simulink model "quaternion_differentiation_test"  (R2016a)
settings: Solver=ode4  StartTime=0.0  StopTime=10.0  FixedStep=0.01  RelTol=1e-3
libraries: aerolibtransform2 x3
settings Model: Creator=PD Banneheka  LastModifiedBy=PD Banneheka
settings GRTTargetCC: GeneratePreprocessorConditionals=Use local settings

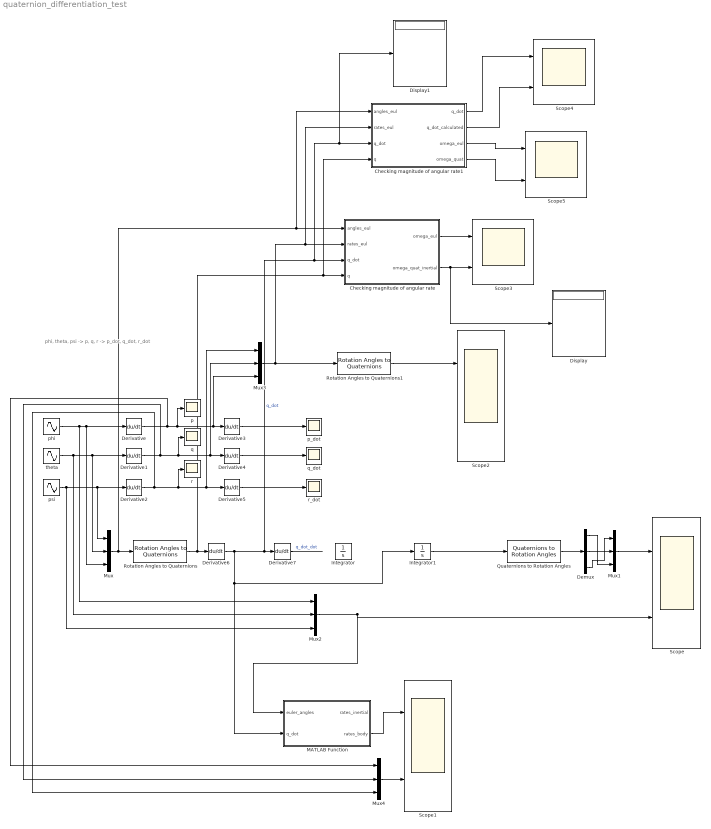
== system quaternion_differentiation_test ==
  note: phi, theta, psi -> p, q, r -> p_dot, q_dot, r_dot
  Checking magnitude of angular rate : MATLAB Function  TreatAsAtomicUnit=on
  Checking magnitude of angular rate1 : MATLAB Function  TreatAsAtomicUnit=on
  Demux : Demux  Outputs=3
  Derivative{,1..7} (8 alike) : Derivative
  Display : Display
  Display1 : Display
  Integrator : Integrator
  Integrator1 : Integrator
  MATLAB Function : MATLAB Function  TreatAsAtomicUnit=on
  Mux{,1..4} (5 alike) : Mux  Inputs=3
  Quaternions to Rotation Angles : aerolibtransform2/Quaternions to Rotation Angles  rotationOrder=ZYX
  Rotation Angles to Quaternions : aerolibtransform2/Rotation Angles to Quaternions  rotationOrder=ZYX
  Rotation Angles to Quaternions1 : aerolibtransform2/Rotation Angles to Quaternions  rotationOrder=ZYX
  Scope{,1..5} (6 alike) : Scope  NumInputPorts=2
  p : Scope
  p_dot : Scope
  phi : Sin  SampleTime=0
  psi : Sin  SampleTime=0
  q : Scope
  q_dot : Scope
  r : Scope
  r_dot : Scope
  theta : Sin  SampleTime=0
  wires:
  phi/1 -> Mux2/1, Mux/3, Derivative/1
  theta/1 -> Mux2/2, Mux/2, Derivative1/1
  psi/1 -> Mux2/3, Derivative2/1, Mux/1
  Derivative3/1 -> p_dot/1
  Derivative4/1 -> q_dot/1
  Derivative5/1 -> r_dot/1
  Mux/1 -> Checking magnitude of angular rate1/1(angles_eul), Checking magnitude of angular rate/1(angles_eul), Rotation Angles to Quaternions/1
  Quaternions to Rotation Angles/1 -> Demux/1
  Demux/1 -> Mux1/3
  Demux/2 -> Mux1/2
  Demux/3 -> Mux1/1
  Mux1/1 -> Scope/1
  Mux2/1 -> MATLAB Function/1(euler_angles), Scope/2
  Mux4/1 -> Scope1/2
  MATLAB Function/2(rates_body) -> Scope1/1
  Derivative/1 -> p/1, Mux3/3, Derivative3/1, Mux4/1
  Derivative1/1 -> q/1, Derivative4/1, Mux3/2, Mux4/2
  Derivative2/1 -> Mux4/3, r/1, Derivative5/1, Mux3/1
  Rotation Angles to Quaternions1/1 -> Scope2/1
  Derivative7/1 -> ?  "q_dot_dot"
  Derivative6/1 -> MATLAB Function/2(q_dot), Integrator1/1, Display1/1, Checking magnitude of angular rate1/3("q_dot "), Checking magnitude of angular rate/3(q_dot), Derivative7/1  "q_dot"
  Rotation Angles to Quaternions/1 -> Derivative6/1, Checking magnitude of angular rate1/4(q), Checking magnitude of angular rate/4(q)
  Integrator1/1 -> Quaternions to Rotation Angles/1
  Mux3/1 -> Checking magnitude of angular rate1/2(rates_eul), Checking magnitude of angular rate/2(rates_eul), Rotation Angles to Quaternions1/1
  Checking magnitude of angular rate/2(omega_quat_inertial) -> Display/1, Scope3/2
  Checking magnitude of angular rate/1(omega_eul) -> Scope3/1
  Checking magnitude of angular rate1/1(q_dot) -> Scope4/1
  Checking magnitude of angular rate1/2(q_dot_calculated) -> Scope4/2
  Checking magnitude of angular rate1/3(omega_eul) -> Scope5/1
  Checking magnitude of angular rate1/4(omega_quat) -> Scope5/2

== matlab function quaternion_differentiation_test/Checking magnitude of angular rate ==
  data: angles_eul input; rates_eul input; omega_eul output; q_dot input; omega_quat_inertial output; q input
function [omega_eul,omega_quat_inertial]= fcn(angles_eul,rates_eul,q_dot,q)
% Checking angular rate
% https://math.stackexchange.com/questions/1792826/estimate-angular-velocity-and-acceleration-from-a-sequence-of-rotations

% Angular rate magnitude using Euler rates
% omega_eul = sqrt(rates_eul(1)^2 + rates_eul(2)^2 + rates_eul(3)^2);
omega_eul = rates_eul;

% From website: omega = 2*q_dot*pinv(q)
% omega_quat = 2*q_dot'*quatinv(q')';
omega_quat = 2*quatmultiply(q_dot',quatinv(q'));

%% Transformation from NASA
% Original axes : inertial/wind/Earth/reference
% Final axes    : body

psi = angles_eul(1); % Yaw angle (first rotation, about z axis)
theta = angles_eul(2); % Pitch angle (second rotation, about y axis)
phi = angles_eul(3); % Roll angle (third rotation, about x axis)

S1 = sin(psi);
C1 = cos(psi);
S2 = sin(theta);
C2 = cos(theta);
S3 = sin(phi);
C3 = cos(phi);
    
M = [   C1*C2               C1*S2*S3-S1*C3      C1*S2*C3+S1*S3
        S1*C2               S1*S2*S3+C1*C3      S1*S2*C3-C1*S3
        -S2                 C2*S3               C2*C3           ]; % x0 = M * x3
    
% omega_quat_inertial = M*omega_quat(2:4)';
omega_quat_inertial = omega_quat(2:4)';

== matlab function quaternion_differentiation_test/MATLAB Function ==
  data: euler_angles input; rates_inertial output; q_dot input; rates_body output
function [rates_inertial,rates_body]= fcn(euler_angles,q_dot)
% From NASA transformation equations:

phi = euler_angles(1);
theta = euler_angles(2);
psi = euler_angles(3);

theta1 = psi;
theta2 = theta;
theta3 = phi;

q0 = +sin(theta1/2)*sin(theta2/2)*sin(theta3/2)+cos(theta1/2)*cos(theta2/2)*cos(theta3/2);
q1 = -sin(theta1/2)*sin(theta2/2)*cos(theta3/2)+sin(theta3/2)*cos(theta1/2)*cos(theta2/2);
q2 = +sin(theta1/2)*sin(theta3/2)*cos(theta2/2)+sin(theta2/2)*cos(theta1/2)*cos(theta3/2);
q3 = +sin(theta1/2)*cos(theta2/2)*cos(theta3/2)-sin(theta2/2)*sin(theta3/2)*cos(theta1/2);

E = [  -q1     q0      -q3     q2
    -q2     q3      q0      -q1
    -q3     -q2     q1      q0  ];

E_dash = [  	-q1     q0      q3      -q2
                -q2     -q3     q0      q1
                -q3     q2      -q1     q0  ];
            
A_b2i = E*transpose(E_dash); % Transforms to initial axes from final axes
            

q0_dot = q_dot(1);
q1_dot = q_dot(2);
q2_dot = q_dot(3);
q3_dot = q_dot(4);

omega_dasha = 2*E_dash*[	q0_dot
                            q1_dot
                            q2_dot
                            q3_dot     ];
                        
p_body = omega_dasha(1);
q_body = omega_dasha(2);
r_body = omega_dasha(3);

rates_inertial = A_b2i*[p_body;q_body;r_body];
rates_body = [p_body;q_body;r_body];

== matlab function quaternion_differentiation_test/Checking magnitude of angular rate1 ==
  data: angles_eul input; rates_eul input; q_dot output; q_dot input; q_dot_calculated output; q input; omega_eul output; omega_quat output
function [q_dot,q_dot_calculated,omega_eul,omega_quat]= fcn(angles_eul,rates_eul,q_dot,q)

% http://stackoverflow.com/questions/23503151/how-to-update-quaternion-based-on-3d-gyro-data

% From website: q_dot = 0.5*q*w
% rate of change quaternion  = q_dot
% quaternion = q
% gyro quaternion = w = [0,gyrox,gyroy,gyroz]

q_dot_calculated = 0.5*quatmultiply(q',[0;rates_eul(1);rates_eul(2);rates_eul(3)]')';

% Angular rate magnitude using Euler rates
% omega_eul = sqrt(rates_eul(1)^2 + rates_eul(2)^2 + rates_eul(3)^2);
omega_eul = rates_eul;

% From website: omega = 2*q_dot*pinv(q)
% omega_quat = 2*q_dot'*quatinv(q')';
omega_quat = 2*quatmultiply(q_dot_calculated',quatinv(q'));
